simulink model "sandbox"  (R2020a)
settings: Solver=VariableStepAuto  StartTime=0.0  StopTime=2e5  RelTol=1e-3
undefined symbols (not defined in the file): agnostic_lqe_params, lqe_params, LQR_params, LQRAgnostic_params, MPC_type, MPCDiscrete_function_parameters, MPCDiscreteAgnostic_function_parameters, MPCDiscreteDiffIntegralAgnostic_function_parameters, original_lqe_params, original_LQR_params, reg
libraries: cstblocks x11
settings Model: SimulationMode=accelerator  Creator=jornbh  LastModifiedBy=jorn
settings OptimizationCC: EfficientMapNaN2IntZero=off
settings HardwareCC: TargetBitPerLong=64  TargetBitPerPointer=64  TargetBitPerSizeT=64  TargetBitPerPtrDiffT=64  TargetLongLongMode=on  TargetIntDivRoundTo=Zero  TargetEndianess=LittleEndian  TargetWordSize=64  TargetHWDeviceType=MATLAB Host  ProdEqTarget=off
settings CodeAppCC: MaxIdLength=128
settings GRTTargetCC: GRTInterface=on  UseToolchainInfoCompliant=off

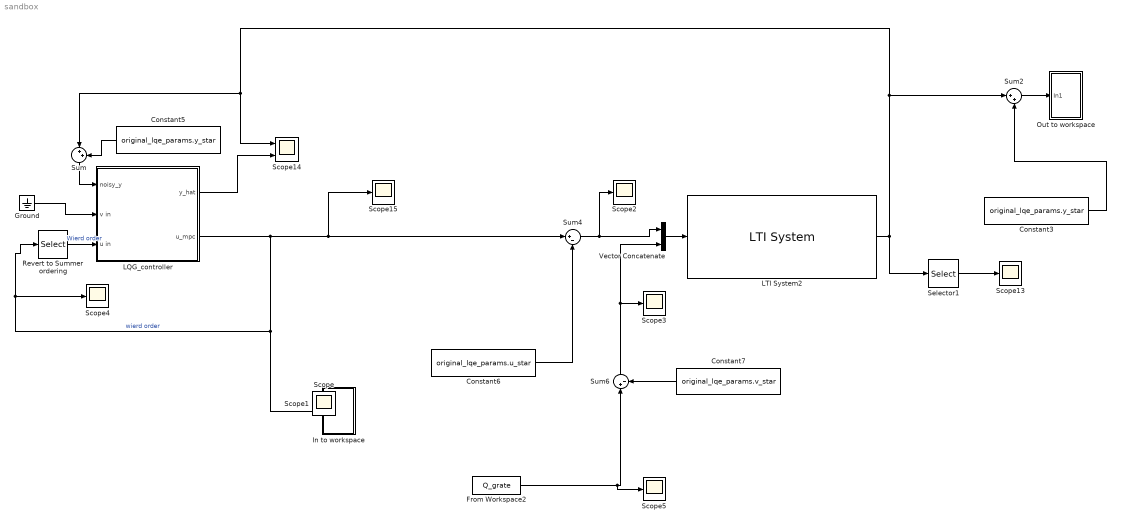
== system sandbox ==
  Constant3 : Constant  Value=original_lqe_params.y_star
  Constant5 : Constant  Value=original_lqe_params.y_star
  Constant6 : Constant  Value=original_lqe_params.u_star
  Constant7 : Constant  Value=original_lqe_params.v_star
  From Workspace2 : FromWorkspace  VariableName=Q_grate  OutputAfterFinalValue=Holding final value
  Ground : Ground
  In to workspace : Subsystem
  LQG_controller : Subsystem
  LTI System2 : cstblocks/LTI System  sys=full_estimated_plant  IC=[]
  Out to workspace : Subsystem
  Revert to Summer ordering : Selector  InputPortWidth=4  IndexOptions=Index vector (dialog)  Indices=[1 3 4 2]  OutputSizes=1
  Scope{,1..5,13,15} (8 alike) : Scope
  Scope14 : Scope  NumInputPorts=2
  Selector1 : Selector  InputPortWidth=3  IndexOptions=Index vector (dialog)  Indices=1:2  OutputSizes=1
  Sum : Sum  Inputs=|++
  Sum2 : Sum  Inputs=|++
  Sum4 : Sum  Inputs=|+-
  Sum6 : Sum  Inputs=|+-
  Vector Concatenate : Concatenate
  wires:
  LTI System2/1 -> Sum2/1, Sum/1, Scope14/1, Selector1/1
  Selector1/1 -> Scope13/1
  LQG_controller/1(y_hat) -> Scope14/2
  Ground/1 -> LQG_controller/2(v in)
  Constant3/1 -> Sum2/2
  Sum2/1 -> Out to workspace/1(In1)
  LQG_controller/2(u_mpc) -> In to workspace/1(u_mpc), Revert to Summer ordering/1, Scope4/1, Sum4/1, Scope15/1  "wierd order"
  Sum4/1 -> Scope2/1, Vector Concatenate/1
  Vector Concatenate/1 -> LTI System2/1
  Sum6/1 -> Scope3/1, Vector Concatenate/2
  Sum/1 -> LQG_controller/1(noisy_y)
  Constant5/1 -> Sum/2
  Constant6/1 -> Sum4/2
  From Workspace2/1 -> Scope5/1, Sum6/1
  Constant7/1 -> Sum6/2
  Revert to Summer ordering/1 -> LQG_controller/3(u in)  "Wierd order"

== system sandbox/In to workspace ==
  u_mpc : Inport
  Demux1 : Demux
  To Workspace4 : ToWorkspace  VariableName=simout_F_w  SaveFormat=Timeseries  SampleTime=-1
  To Workspace5 : ToWorkspace  VariableName=simout_F_aI  SaveFormat=Timeseries  SampleTime=-1
  To Workspace6 : ToWorkspace  VariableName=simout_F_aII  SaveFormat=Timeseries  SampleTime=-1
  To Workspace7 : ToWorkspace  VariableName=simout_v_grate  SaveFormat=Timeseries  SampleTime=-1
  wires:
  Demux1/3 -> To Workspace5/1
  Demux1/1 -> To Workspace6/1
  u_mpc/1 -> Demux1/1
  Demux1/2 -> To Workspace4/1
  Demux1/4 -> To Workspace7/1

== system sandbox/LQG_controller ==
  noisy_y : Inport  OutDataTypeStr=double
  v in : Inport  Port=2
  u in : Inport  Port=3
  Demux : Demux  Outputs=3
  MPC_subsystem : Subsystem
      settings: PortSchema="{\"entries\":[{\"content\":{\"sides\":[{\"content\":{\"connectorIds\":[\"In1\",\"In2\",\"In3\"]},\"type\":\"ConnectorPlacement.EquallySpacedRectSide\",\"uuid\":\"7a72dc7f-38c0-42c0-80ed-1e6801fa5538\"},{\"content\":{\"connectorIds\":[\"Out1\",\"Out2\",\"Out3\",\"Out4\",\"Out5\"],\"side\":\"RIGHT\"},\"type\":\"ConnectorPlacement.EquallySpacedRectSide\",\"uuid\":\"3b96338e-56f2-4c6d-b025-d8deebb787e0\"},{\"content\":{\"connectorIds\":[],\"side\":\"TOP\"},\"type\":\"ConnectorPlacement.EquallySpacedRectSide\",\"uuid\":\"204ca672-7e69-45d1-bd78-35e421377db1\"},{\"content\":{\"connectorIds\":[\"In4\",\"In5\"],\"side\":\"BOTTOM\"},\"type\":\"ConnectorPlacement.EquallySpacedRectSide\",\"uuid\":\"d178d855-840b-4794-a5e2-c07226929ecd\"}]},\"type\":\"ConnectorPlacement.EquallySpacedConnector\",\"uuid\":\"1be467ef-13fc-4acb-88f5-eb362f838469\"}],\"packageUris\":[\"http://schema.mathworks.com/mf0/Connector/19700101\"],\"version\":\"1.0\"}"
  Mux : Mux
  y_hat : Outport
  u_mpc : Outport  Port=2
  wires:
  u in/1 -> MPC_subsystem/4(used_inputs)
  v in/1 -> MPC_subsystem/5("\"Measured\" disturbances")
  MPC_subsystem/1(F_aII_MPC) -> Mux/1
  MPC_subsystem/2(F_aI_MPC) -> Mux/3
  MPC_subsystem/3(v_grate_MPC) -> Mux/4
  MPC_subsystem/4(F_w_MPC) -> Mux/2
  Mux/1 -> u_mpc/1
  MPC_subsystem/5(y_hat) -> y_hat/1
  Demux/2 -> MPC_subsystem/1(F_O2_in)
  Demux/1 -> MPC_subsystem/2(F_st_in)
  Demux/3 -> MPC_subsystem/3(HHV_in)
  noisy_y/1 -> Demux/1

== system sandbox/Out to workspace ==
  In1 : Inport
  Demux : Demux  Outputs=3
  To Workspace1 : ToWorkspace  VariableName=simout_HHV  SaveFormat=Timeseries  SampleTime=-1
  To Workspace2 : ToWorkspace  VariableName=simout_F_O2  SaveFormat=Timeseries  SampleTime=-1
  To Workspace3 : ToWorkspace  VariableName=simout_F_st  SaveFormat=Timeseries  SampleTime=-1
  wires:
  Demux/1 -> To Workspace3/1
  Demux/2 -> To Workspace2/1
  Demux/3 -> To Workspace1/1
  In1/1 -> Demux/1

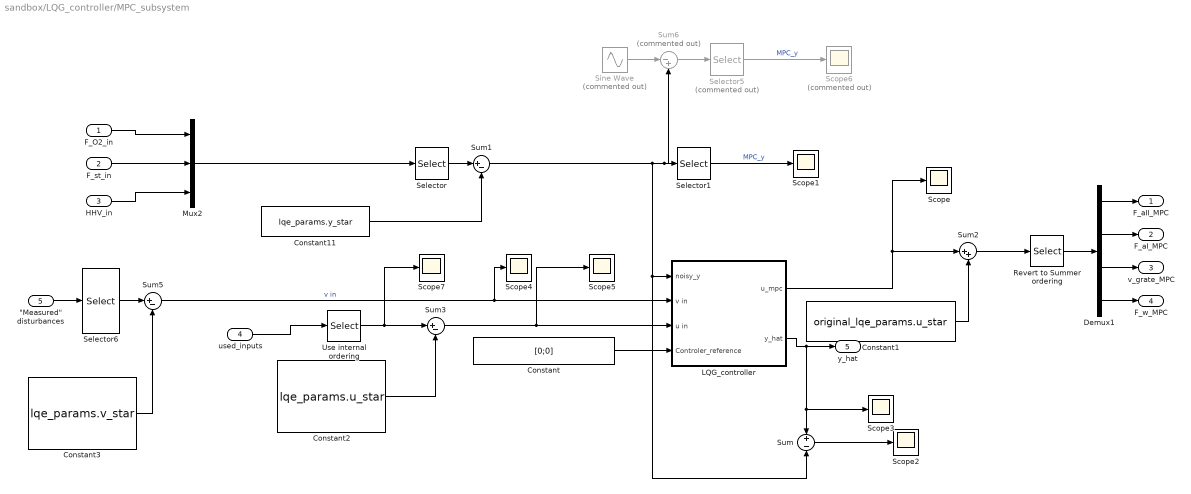
== system sandbox/LQG_controller/MPC_subsystem ==
  F_O2_in : Inport
  F_st_in : Inport  Port=2
  HHV_in : Inport  Port=3
  used_inputs : Inport  Port=4
  "\"Measured\" disturbances" : Inport  Port=5
  Constant : Constant  Value=[0;0]
  Constant1 : Constant  Value=original_lqe_params.u_star
  Constant11 : Constant  Value=lqe_params.y_star
  Constant2 : Constant  Value=lqe_params.u_star
  Constant3 : Constant  Value=lqe_params.v_star
  Demux1 : Demux
  LQG_controller : Subsystem
  Mux2 : Mux  Inputs=3
  Revert to Summer ordering : Selector  InputPortWidth=4  IndexOptions=Index vector (dialog)  Indices=[1 3 4 2]  OutputSizes=1
  Scope{,1..5,7} (7 alike) : Scope
  Scope6 : Scope  Commented=on
  Selector : Selector  InputPortWidth=3  IndexOptions=Index vector (dialog)  Indices=[2 1 3]  OutputSizes=1
  Selector1 : Selector  InputPortWidth=3  IndexOptions=Index vector (dialog)  Indices=1:2  OutputSizes=1
  Selector5 : Selector  Commented=on  InputPortWidth=3  IndexOptions=Index vector (dialog)  Indices=1:2  OutputSizes=1
  Selector6 : Selector  InputPortWidth=5  IndexOptions=Index vector (dialog)  Indices=original_lqe_params.disturbance_measurement_indecies  OutputSizes=1
  Sine Wave : Sin  Commented=on  Amplitude=reg.include_noise * 1e-3  SampleTime=0
  Sum : Sum  Inputs=+-
  Sum1 : Sum  Inputs=|+-
  Sum2 : Sum  Inputs=|++
  Sum3 : Sum  Inputs=|+-
  Sum5 : Sum  Inputs=|+-
  Sum6 : Sum  Commented=on  Inputs=|-+
  Use internal ordering : Selector  InputPortWidth=4  IndexOptions=Index vector (dialog)  Indices=[1 4 2 3]  OutputSizes=1
  F_aII_MPC : Outport
  F_aI_MPC : Outport  Port=2
  v_grate_MPC : Outport  Port=3
  F_w_MPC : Outport  Port=4
  y_hat : Outport  Port=5
  wires:
  Demux1/1 -> F_aII_MPC/1
  Demux1/3 -> v_grate_MPC/1
  Constant/1 -> LQG_controller/4(Controler_reference)
  Demux1/2 -> F_aI_MPC/1
  HHV_in/1 -> Mux2/3
  F_O2_in/1 -> Mux2/1
  F_st_in/1 -> Mux2/2
  Constant11/1 -> Sum1/2
  Demux1/4 -> F_w_MPC/1
  Sum2/1 -> Revert to Summer ordering/1
  Revert to Summer ordering/1 -> Demux1/1
  Selector/1 -> Sum1/1
  Selector1/1 -> Scope1/1  "MPC_y"
  Sum/1 -> Scope2/1
  Sum1/1 -> LQG_controller/1(noisy_y), Sum/2, Sum6/2, Selector1/1
  used_inputs/1 -> Use internal ordering/1
  Sum3/1 -> LQG_controller/3(u in), Scope5/1
  Constant2/1 -> Sum3/2
  Use internal ordering/1 -> Scope7/1, Sum3/1
  Mux2/1 -> Selector/1
  Selector5/1 -> Scope6/1  "MPC_y"
  Sine Wave/1 -> Sum6/1
  Sum6/1 -> Selector5/1
  "\"Measured\" disturbances"/1 -> Selector6/1
  Constant3/1 -> Sum5/2
  Sum5/1 -> LQG_controller/2(v in), Scope4/1  "v in"
  Selector6/1 -> Sum5/1
  Constant1/1 -> Sum2/2
  LQG_controller/2(y_hat) -> y_hat/1, Scope3/1, Sum/1
  LQG_controller/1(u_mpc) -> Scope/1, Sum2/1

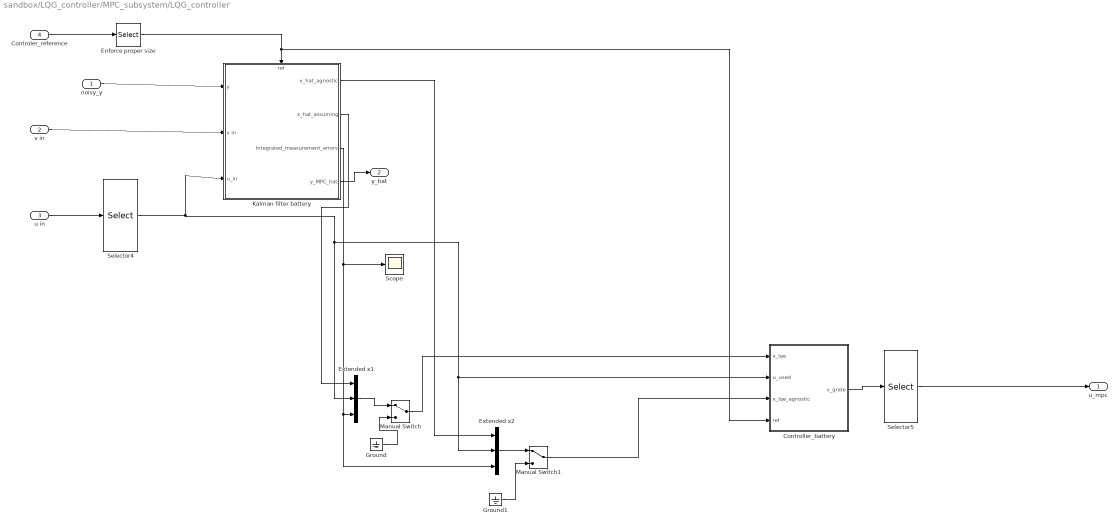
== system sandbox/LQG_controller/MPC_subsystem/LQG_controller ==
  noisy_y : Inport  OutDataTypeStr=double
  v in : Inport  Port=2
  u in : Inport  Port=3
  Controler_reference : Inport  Port=4  OutDataTypeStr=double
  Controller_battery : Subsystem
  Enforce proper size : Selector  InputPortWidth=original_LQR_params.N_refs  IndexOptions=Index vector (dialog)  Indices=1:original_LQR_params.N_refs  OutputSizes=1
  Extended x1 : Concatenate  NumInputs=3
  Extended x2 : Concatenate  NumInputs=3
  Ground : Ground
  Ground1 : Ground
  Kalman filter battery : Subsystem
      settings: PortSchema="{\"entries\":[{\"content\":{\"sides\":[{\"content\":{\"connectorIds\":[\"In1\",\"In2\",\"In3\"]},\"type\":\"ConnectorPlacement.EquallySpacedRectSide\",\"uuid\":\"1c993a74-2ebc-4ff1-8a36-810b6615b91b\"},{\"content\":{\"connectorIds\":[\"Out1\",\"Out2\",\"Out3\",\"Out4\"],\"side\":\"RIGHT\"},\"type\":\"ConnectorPlacement.EquallySpacedRectSide\",\"uuid\":\"f47ce850-e8b0-4437-a8da-01c6ea316d70\"},{\"content\":{\"connectorIds\":[],\"side\":\"TOP\"},\"type\":\"ConnectorPlacement.EquallySpacedRectSide\",\"uuid\":\"49075f58-3726-424f-842a-93e04b24d953\"},{\"content\":{\"connectorIds\":[\"In4\"],\"side\":\"BOTTOM\"},\"type\":\"ConnectorPlacement.EquallySpacedRectSide\",\"uuid\":\"0a8cab2c-6cc5-4573-a1bf-983f74a1ee29\"}]},\"type\":\"ConnectorPlacement.EquallySpacedConnector\",\"uuid\":\"113553bc-ba05-4a25-98d3-042b5b48218e\"}],\"packageUris\":[\"http://schema.mathworks.com/mf0/Connector/19700101\"],\"version\":\"1.0\"}"
  Manual Switch : ManualSwitch
  Manual Switch1 : ManualSwitch
  Scope : Scope
  Selector4 : Selector  InputPortWidth=4  IndexOptions=Index vector (dialog)  Indices=1:4  OutputSizes=1
  Selector5 : Selector  InputPortWidth=4  IndexOptions=Index vector (dialog)  Indices=1:4  OutputSizes=1
  u_mpc : Outport
  y_hat : Outport  Port=2
  wires:
  Controler_reference/1 -> Enforce proper size/1
  u in/1 -> Selector4/1
  Enforce proper size/1 -> Controller_battery/4(ref), Kalman filter battery/4(ref)
  Kalman filter battery/2(Integrated_measurement_errors) -> Extended x2/3, Extended x1/3, Scope/1
  noisy_y/1 -> Kalman filter battery/3(y)
  Kalman filter battery/1(y_MPC_hat) -> y_hat/1
  Selector5/1 -> u_mpc/1
  Selector4/1 -> Extended x1/2, Extended x2/2, Controller_battery/2(u_used), Kalman filter battery/1(u_in)
  Controller_battery/1(v_grate) -> Selector5/1
  v in/1 -> Kalman filter battery/2(v in)
  Kalman filter battery/4(x_hat_agnostic) -> Extended x2/1
  Manual Switch/1 -> Controller_battery/1(x_lqe)
  Manual Switch1/1 -> Controller_battery/3(x_lqe_agnostic)
  Kalman filter battery/3(x_hat_assuming) -> Extended x1/1
  Extended x1/1 -> Manual Switch/1
  Extended x2/1 -> Manual Switch1/1
  Ground/1 -> Manual Switch/2
  Ground1/1 -> Manual Switch1/2

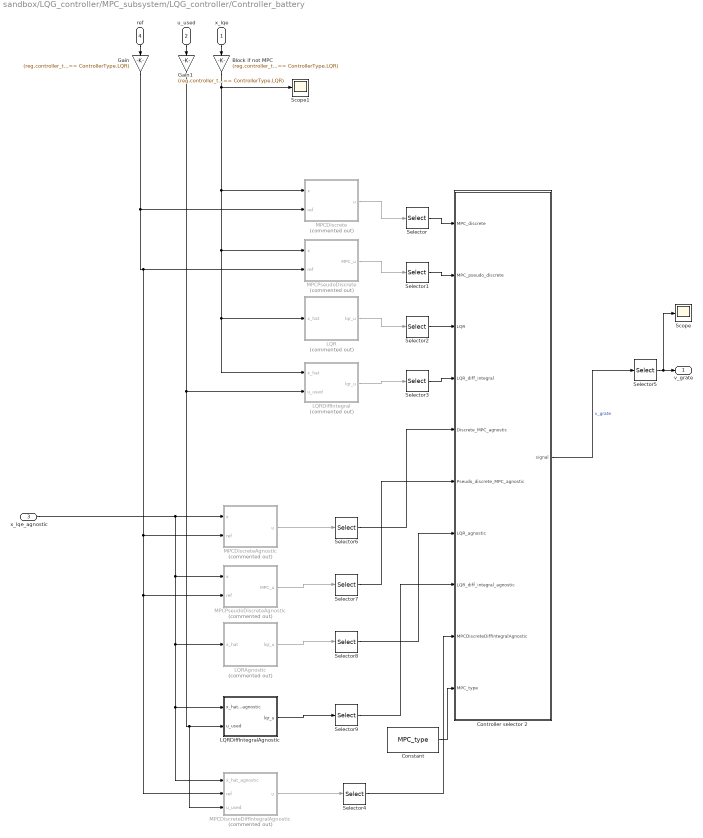
== system sandbox/LQG_controller/MPC_subsystem/LQG_controller/Controller_battery ==
  x_lqe : Inport
  u_used : Inport  Port=2
  x_lqe_agnostic : Inport  Port=3
  ref : Inport  Port=4
  Block if not MPC : Gain  Gain=(reg.controller_type == ControllerType.MPC)|| (reg.controller_type == ControllerType.LQR)
  Constant : Constant  Value=MPC_type
  Controller selector 2 : MATLAB Function  TreatAsAtomicUnit=on
  Gain : Gain  Gain=(reg.controller_type == ControllerType.MPC)|| (reg.controller_type == ControllerType.LQR)
  Gain1 : Gain  Gain=(reg.controller_type == ControllerType.MPC)|| (reg.controller_type == ControllerType.LQR)
  LQR : Subsystem  Commented=on
  LQRAgnostic : Subsystem  Commented=on
  LQRDiffIntegral : Subsystem  Commented=on
  LQRDiffIntegralAgnostic : Subsystem
  MPCDiscrete : Subsystem  Commented=on
  MPCDiscreteAgnostic : Subsystem  Commented=on
  MPCDiscreteDiffIntegralAgnostic : Subsystem  Commented=on
  MPCPseudoDiscrete : Subsystem  Commented=on
  MPCPseudoDiscreteAgnostic : Subsystem  Commented=on
  Scope : Scope
  Scope1 : Scope
  Selector{,1..9} (10 alike) : Selector  InputPortWidth=4  IndexOptions=Index vector (dialog)  Indices=1:4  OutputSizes=1
  v_grate : Outport
  wires:
  MPCPseudoDiscrete/1(MPC_u) -> Selector1/1
  LQR/1(lqr_u) -> Selector2/1
  MPCDiscrete/1(u) -> Selector/1
  LQRDiffIntegral/1(lqr_u) -> Selector3/1
  Controller selector 2/1(signal) -> Selector5/1  "v_grate"
  u_used/1 -> Gain1/1
  ref/1 -> Gain/1
  x_lqe/1 -> Block if not MPC/1
  Selector/1 -> Controller selector 2/1(MPC_discrete)
  Selector1/1 -> Controller selector 2/2(MPC_pseudo_discrete)
  Selector2/1 -> Controller selector 2/3(LQR)
  Selector3/1 -> Controller selector 2/4(LQR_diff_integral)
  Constant/1 -> Controller selector 2/10(MPC_type)
  Selector5/1 -> Scope/1, v_grate/1
  MPCDiscreteAgnostic/1(u) -> Selector6/1
  LQRDiffIntegralAgnostic/1(lqr_u) -> Selector9/1
  LQRAgnostic/1(lqr_u) -> Selector8/1
  MPCPseudoDiscreteAgnostic/1(MPC_u) -> Selector7/1
  Selector6/1 -> Controller selector 2/5(Discrete_MPC_agnostic)
  Selector9/1 -> Controller selector 2/8(LQR_diff_integral_agnostic)
  Selector7/1 -> Controller selector 2/6(Pseudo_discrete_MPC_agnostic)
  Selector8/1 -> Controller selector 2/7(LQR_agnostic)
  Gain/1 -> MPCDiscreteDiffIntegralAgnostic/2(ref), MPCPseudoDiscreteAgnostic/2(ref), MPCDiscreteAgnostic/2(ref), MPCPseudoDiscrete/2(ref), MPCDiscrete/2(ref)
  Block if not MPC/1 -> Scope1/1, LQRDiffIntegral/1(x_hat), LQR/1(x_hat), MPCPseudoDiscrete/1(x), MPCDiscrete/1(x)
  x_lqe_agnostic/1 -> MPCPseudoDiscreteAgnostic/1(x), LQRAgnostic/1(x_hat), MPCDiscreteDiffIntegralAgnostic/1(x_hat_agnostic), LQRDiffIntegralAgnostic/1(x_hat_agnostic), MPCDiscreteAgnostic/1(x)
  MPCDiscreteDiffIntegralAgnostic/1(u) -> Selector4/1
  Selector4/1 -> Controller selector 2/9(MPCDiscreteDiffIntegralAgnostic)
  Gain1/1 -> MPCDiscreteDiffIntegralAgnostic/3(u_used), LQRDiffIntegralAgnostic/2(u_used), LQRDiffIntegral/2(u_used)

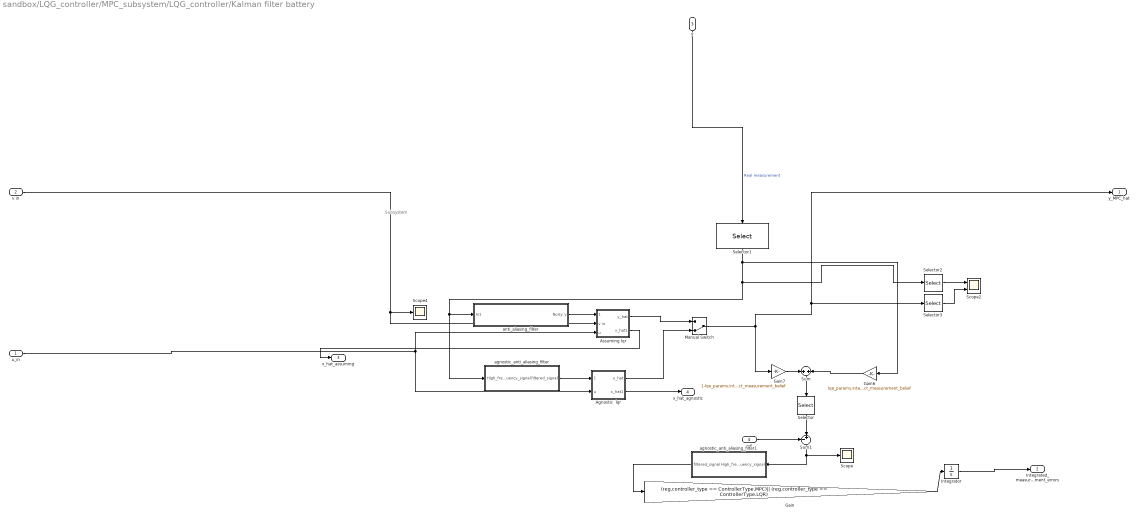
== system sandbox/LQG_controller/MPC_subsystem/LQG_controller/Kalman filter battery ==
  note: Subsystem
  u_in : Inport
  v in : Inport  Port=2
  y : Inport  Port=3
  ref : Inport  Port=4
  Agnostic  lqr : Subsystem
  Assuming lqr : Subsystem
  Gain : Gain  Gain=(reg.controller_type == ControllerType.MPC)|| (reg.controller_type == ControllerType.LQR)
  Gain6 : Gain  Gain=lqe_params.integrator_direct_measurement_belief
  Gain7 : Gain  Gain=1-lqe_params.integrator_direct_measurement_belief
  Integrator : Integrator
  Manual Switch : ManualSwitch  CurrentSetting=0
  Scope : Scope
  Scope2 : Scope  NumInputPorts=2
  Scope4 : Scope
  Selector : Selector  InputPortWidth=3  IndexOptions=Index vector (dialog)  Indices=1:2  OutputSizes=1
  Selector1 : Selector  InputPortWidth=3  IndexOptions=Index vector (dialog)  Indices=1:3  OutputSizes=1
  Selector2 : Selector  InputPortWidth=3  IndexOptions=Index vector (dialog)  Indices=1:2  OutputSizes=1
  Selector3 : Selector  InputPortWidth=3  IndexOptions=Index vector (dialog)  Indices=1:2  OutputSizes=1
  Sum : Sum
  Sum1 : Sum  Inputs=-+|
  agnostic_anti_aliasing_filter : Subsystem
  agnostic_anti_aliasing_filter1 : Subsystem
  anti_aliasing_filter : Subsystem
  y_MPC_hat : Outport
  Integrated_measurement_errors : Outport  Port=2
  x_hat_assuming : Outport  Port=3
  x_hat_agnostic : Outport  Port=4
  wires:
  y/1 -> Selector1/1  "Real measurement"
  Manual Switch/1 -> y_MPC_hat/1, Selector3/1, Gain7/1
  Integrator/1 -> Integrated_measurement_errors/1
  Assuming lqr/2(x_hat1) -> x_hat_assuming/1
  Agnostic  lqr/2(x_hat1) -> x_hat_agnostic/1
  Selector/1 -> Sum1/2
  Gain/1 -> Integrator/1
  Assuming lqr/1(y_hat) -> Manual Switch/1
  u_in/1 -> Agnostic  lqr/2(u), Assuming lqr/3(u)
  Gain7/1 -> Sum/1
  ref/1 -> Sum1/1
  Selector1/1 -> anti_aliasing_filter/1(In1), agnostic_anti_aliasing_filter/1(High_frequency_signal), Selector2/1, Gain6/1
  Sum1/1 -> Scope/1, agnostic_anti_aliasing_filter1/1(High_frequency_signal)
  Selector2/1 -> Scope2/1
  v in/1 -> Assuming lqr/2(v in), Scope4/1
  Agnostic  lqr/1(y_hat) -> Manual Switch/2
  Sum/1 -> Selector/1
  Selector3/1 -> Scope2/2
  anti_aliasing_filter/1(Noisy y) -> Assuming lqr/1(Noisy y)
  Gain6/1 -> Sum/2
  agnostic_anti_aliasing_filter/1(filtered_signal) -> Agnostic  lqr/1(Noisy y)
  agnostic_anti_aliasing_filter1/1(filtered_signal) -> Gain/1

== system sandbox/LQG_controller/MPC_subsystem/LQG_controller/Controller_battery/LQR ==
  x_hat : Inport
  LQR : Gain  Gain=-LQR_params.K_lqr  Multiplication=Matrix(K*u)
  LTI System1 : cstblocks/LTI System  sys=original_LQR_params.input_filter  IC=[]
  Scope1 : Scope
  Scope2 : Scope
  lqr_u : Outport
  wires:
  LQR/1 -> LTI System1/1  "lqr_u"
  x_hat/1 -> Scope1/1, LQR/1
  LTI System1/1 -> Scope2/1, lqr_u/1

== system sandbox/LQG_controller/MPC_subsystem/LQG_controller/Controller_battery/LQRAgnostic ==
  x_hat : Inport
  LQR : Gain  Gain=-LQRAgnostic_params.K_lqr  Multiplication=Matrix(K*u)
  LTI System1 : cstblocks/LTI System  sys=original_LQRAgnostic_params.input_filter  IC=[]
  Scope1 : Scope
  Scope2 : Scope
  lqr_u : Outport
  wires:
  LTI System1/1 -> Scope2/1, lqr_u/1
  x_hat/1 -> LQR/1, Scope1/1
  LQR/1 -> LTI System1/1  "lqr_u"

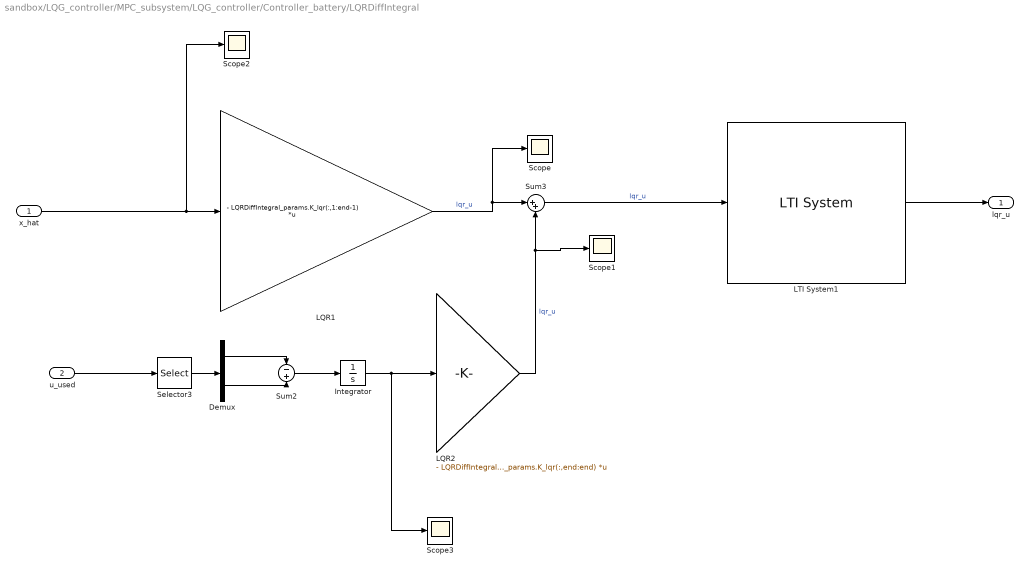
== system sandbox/LQG_controller/MPC_subsystem/LQG_controller/Controller_battery/LQRDiffIntegral ==
  x_hat : Inport
  u_used : Inport  Port=2
  Demux : Demux  Outputs=2
  Integrator : Integrator
  LQR1 : Gain  Gain=- LQRDiffIntegral_params.K_lqr(:,1:end-1)  Multiplication=Matrix(K*u)
  LQR2 : Gain  Gain=- LQRDiffIntegral_params.K_lqr(:,end:end)  Multiplication=Matrix(K*u)
  LTI System1 : cstblocks/LTI System  sys=original_LQRDiffIntegral_params.input_filter  IC=[]
  Scope{,1..3} (4 alike) : Scope
  Selector3 : Selector  InputPortWidth=4  IndexOptions=Index vector (dialog)  Indices=[1 3]  OutputSizes=1
  Sum2 : Sum  Inputs=-+
  Sum3 : Sum  Inputs=|++
  lqr_u : Outport
  wires:
  LQR1/1 -> Scope/1, Sum3/1  "lqr_u"
  u_used/1 -> Selector3/1
  Sum3/1 -> LTI System1/1  "lqr_u"
  Sum2/1 -> Integrator/1
  Demux/2 -> Sum2/2
  Integrator/1 -> Scope3/1, LQR2/1
  Selector3/1 -> Demux/1
  Demux/1 -> Sum2/1
  x_hat/1 -> Scope2/1, LQR1/1
  LQR2/1 -> Scope1/1, Sum3/2  "lqr_u"
  LTI System1/1 -> lqr_u/1

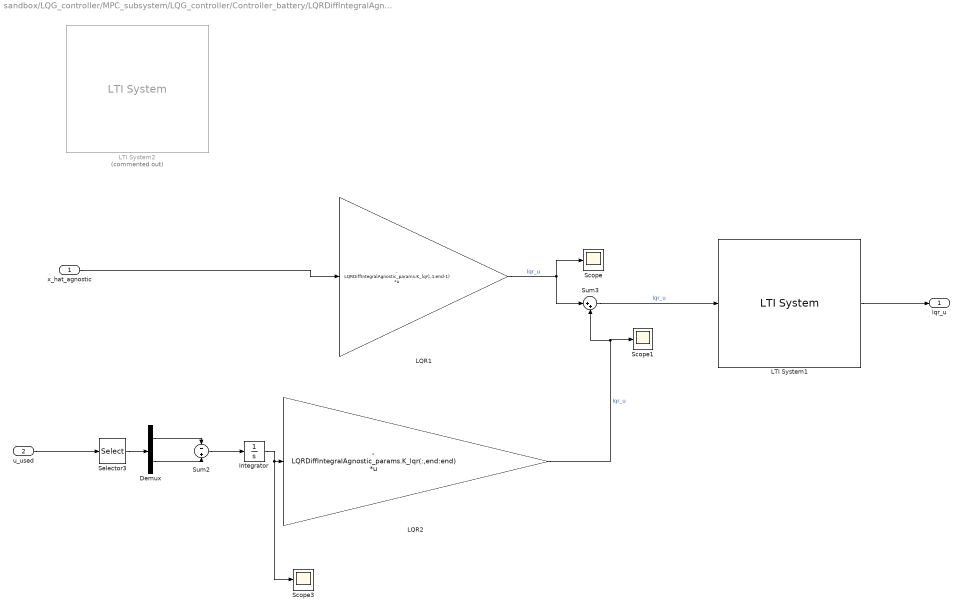
== system sandbox/LQG_controller/MPC_subsystem/LQG_controller/Controller_battery/LQRDiffIntegralAgnostic ==
  x_hat_agnostic : Inport
  u_used : Inport  Port=2
  Demux : Demux  Outputs=2
  Integrator : Integrator
  LQR1 : Gain  Gain=- LQRDiffIntegralAgnostic_params.K_lqr(:,1:end-1)  Multiplication=Matrix(K*u)
  LQR2 : Gain  Gain=- LQRDiffIntegralAgnostic_params.K_lqr(:,end:end)  Multiplication=Matrix(K*u)
  LTI System1 : cstblocks/LTI System  sys=original_LQRDiffIntegralAgnostic_params.input_filter  IC=[]
  LTI System2 : cstblocks/LTI System  Commented=on  sys=original_diff_agnostic_mpc_params.input_filter  IC=[]
  Scope : Scope
  Scope1 : Scope
  Scope3 : Scope
  Selector3 : Selector  InputPortWidth=4  IndexOptions=Index vector (dialog)  Indices=[1 3]  OutputSizes=1
  Sum2 : Sum  Inputs=-+
  Sum3 : Sum  Inputs=|++
  lqr_u : Outport
  wires:
  LQR2/1 -> Sum3/2, Scope1/1  "lqr_u"
  Demux/1 -> Sum2/1
  Selector3/1 -> Demux/1
  Integrator/1 -> Scope3/1, LQR2/1
  Demux/2 -> Sum2/2
  Sum2/1 -> Integrator/1
  Sum3/1 -> LTI System1/1  "lqr_u"
  LQR1/1 -> Sum3/1, Scope/1  "lqr_u"
  LTI System1/1 -> lqr_u/1
  x_hat_agnostic/1 -> LQR1/1
  u_used/1 -> Selector3/1

== system sandbox/LQG_controller/MPC_subsystem/LQG_controller/Controller_battery/MPCDiscrete ==
  x : Inport
  ref : Inport  Port=2
  LTI System1 : cstblocks/LTI System  sys=original_MPCDiscrete_params .input_filter  IC=[]
  MATLAB Function : MATLAB Function  TreatAsAtomicUnit=on
  Memory1 : Memory  InitialCondition=MPCDiscrete_function_parameters.iA  InheritSampleTime=on  LinearizeMemory=on  LinearizeAsDelay=on
  Memory4 : Memory  InheritSampleTime=on  LinearizeMemory=on  LinearizeAsDelay=on
  u : Outport
  wires:
  Memory4/1 -> MATLAB Function/3(u_prev)
  MATLAB Function/2(new_iA) -> Memory1/1
  MATLAB Function/1(u) -> LTI System1/1, Memory4/1
  Memory1/1 -> MATLAB Function/4(iA)
  ref/1 -> MATLAB Function/2(ref)
  x/1 -> MATLAB Function/1(x)
  LTI System1/1 -> u/1

== system sandbox/LQG_controller/MPC_subsystem/LQG_controller/Controller_battery/MPCDiscreteAgnostic ==
  x : Inport
  ref : Inport  Port=2
  LTI System1 : cstblocks/LTI System  sys=original_MPCDiscreteAgnostic_params.input_filter  IC=[]
  MATLAB Function : MATLAB Function  TreatAsAtomicUnit=on
  Memory1 : Memory  InitialCondition=MPCDiscreteAgnostic_function_parameters.iA  InheritSampleTime=on  LinearizeMemory=on  LinearizeAsDelay=on
  Memory4 : Memory  InheritSampleTime=on  LinearizeMemory=on  LinearizeAsDelay=on
  u : Outport
  wires:
  LTI System1/1 -> u/1
  x/1 -> MATLAB Function/1(x)
  ref/1 -> MATLAB Function/2(ref)
  Memory1/1 -> MATLAB Function/4(iA)
  MATLAB Function/1(u) -> Memory4/1, LTI System1/1
  MATLAB Function/2(new_iA) -> Memory1/1
  Memory4/1 -> MATLAB Function/3(u_prev)

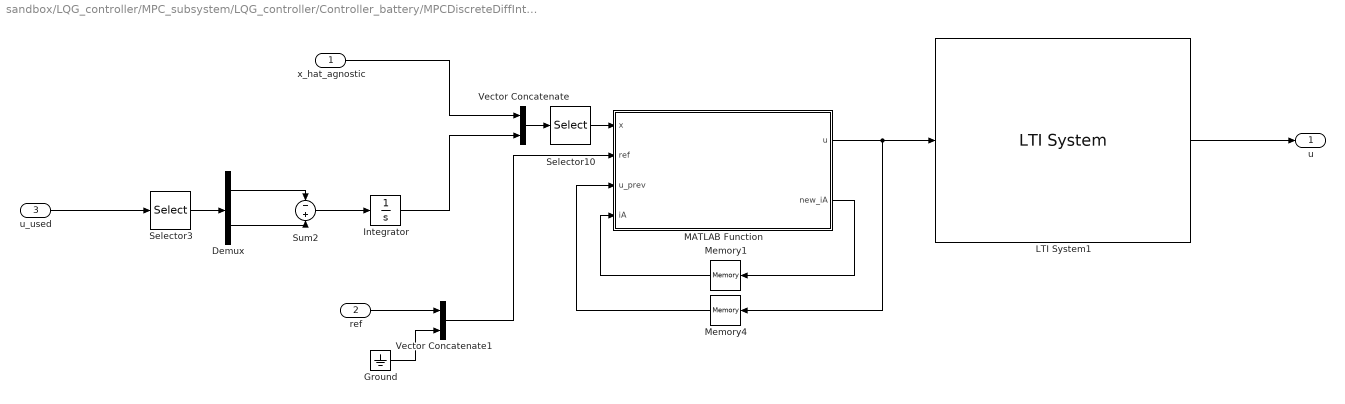
== system sandbox/LQG_controller/MPC_subsystem/LQG_controller/Controller_battery/MPCDiscreteDiffIntegralAgnostic ==
  x_hat_agnostic : Inport
  ref : Inport  Port=2
  u_used : Inport  Port=3
  Demux : Demux  Outputs=2
  Ground : Ground
  Integrator : Integrator
  LTI System1 : cstblocks/LTI System  sys=original_MPCDiscreteAgnostic_params.input_filter  IC=[]
  MATLAB Function : MATLAB Function  TreatAsAtomicUnit=on
  Memory1 : Memory  InitialCondition=MPCDiscreteDiffIntegralAgnostic_function_parameters.iA  InheritSampleTime=on  LinearizeMemory=on  LinearizeAsDelay=on
  Memory4 : Memory  InheritSampleTime=on  LinearizeMemory=on  LinearizeAsDelay=on
  Selector10 : Selector  InputPortWidth=19  IndexOptions=Index vector (dialog)  Indices=1:19  OutputSizes=1
  Selector3 : Selector  InputPortWidth=4  IndexOptions=Index vector (dialog)  Indices=[1 3]  OutputSizes=1
  Sum2 : Sum  Inputs=-+
  Vector Concatenate : Concatenate
  Vector Concatenate1 : Concatenate
  u : Outport
  wires:
  LTI System1/1 -> u/1
  x_hat_agnostic/1 -> Vector Concatenate/1
  Vector Concatenate1/1 -> MATLAB Function/2(ref)
  Memory1/1 -> MATLAB Function/4(iA)
  MATLAB Function/1(u) -> Memory4/1, LTI System1/1
  MATLAB Function/2(new_iA) -> Memory1/1
  Memory4/1 -> MATLAB Function/3(u_prev)
  Selector3/1 -> Demux/1
  Demux/1 -> Sum2/1
  u_used/1 -> Selector3/1
  Demux/2 -> Sum2/2
  Sum2/1 -> Integrator/1
  Integrator/1 -> Vector Concatenate/2
  Vector Concatenate/1 -> Selector10/1
  Selector10/1 -> MATLAB Function/1(x)
  ref/1 -> Vector Concatenate1/1
  Ground/1 -> Vector Concatenate1/2

== system sandbox/LQG_controller/MPC_subsystem/LQG_controller/Controller_battery/MPCPseudoDiscrete ==
  x : Inport
  ref : Inport  Port=2
  Cont mpc : MATLAB Function
  LTI System1 : cstblocks/LTI System  sys=original_MPCPseudoDiscrete_params.input_filter  IC=[]
  MPC_u : Outport
  wires:
  Cont mpc/1(u) -> LTI System1/1  "MPC_u"
  x/1 -> Cont mpc/1(x)
  ref/1 -> Cont mpc/2(ref)
  LTI System1/1 -> MPC_u/1

== system sandbox/LQG_controller/MPC_subsystem/LQG_controller/Controller_battery/MPCPseudoDiscreteAgnostic ==
  x : Inport
  ref : Inport  Port=2
  Cont mpc : MATLAB Function
  LTI System1 : cstblocks/LTI System  sys=original_MPCPseudoDiscreteAgnostic_params.input_filter  IC=[]
  MPC_u : Outport
  wires:
  LTI System1/1 -> MPC_u/1
  ref/1 -> Cont mpc/2(ref)
  x/1 -> Cont mpc/1(x)
  Cont mpc/1(u) -> LTI System1/1  "MPC_u"

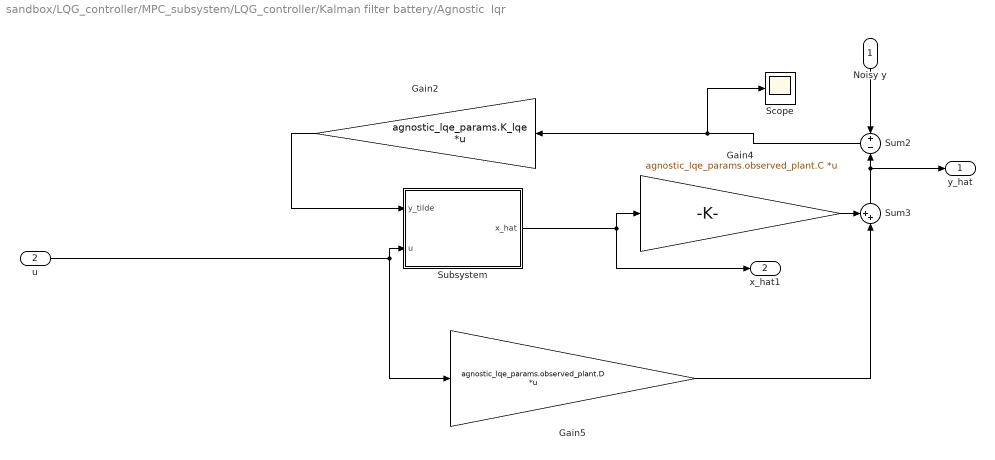
== system sandbox/LQG_controller/MPC_subsystem/LQG_controller/Kalman filter battery/Agnostic  lqr ==
  Noisy y : Inport
  u : Inport  Port=2
  Gain2 : Gain  Gain=agnostic_lqe_params.K_lqe  Multiplication=Matrix(K*u)
  Gain4 : Gain  Gain=agnostic_lqe_params.observed_plant.C  Multiplication=Matrix(K*u)
  Gain5 : Gain  Gain=agnostic_lqe_params.observed_plant.D  Multiplication=Matrix(K*u)
  Scope : Scope
  Subsystem : Subsystem
  Sum2 : Sum  Inputs=+-
  Sum3 : Sum  Inputs=++|
  y_hat : Outport
  x_hat1 : Outport  Port=2
  wires:
  Noisy y/1 -> Sum2/1
  Gain5/1 -> Sum3/2
  Gain4/1 -> Sum3/1
  Sum2/1 -> Gain2/1, Scope/1
  u/1 -> Gain5/1, Subsystem/2(u)
  Sum3/1 -> y_hat/1, Sum2/2
  Subsystem/1(x_hat) -> Gain4/1, x_hat1/1
  Gain2/1 -> Subsystem/1(y_tilde)

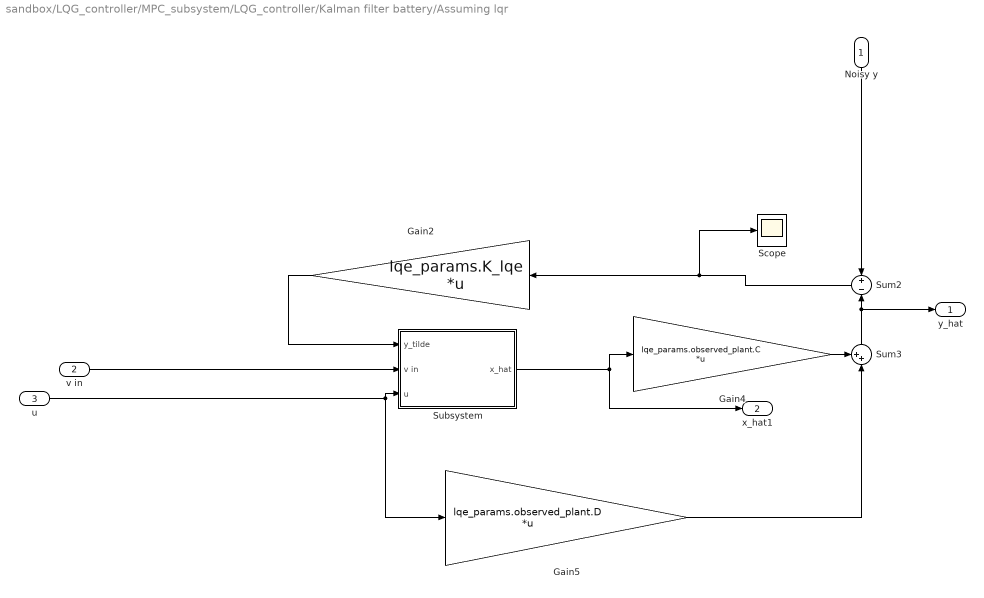
== system sandbox/LQG_controller/MPC_subsystem/LQG_controller/Kalman filter battery/Assuming lqr ==
  Noisy y : Inport
  v in : Inport  Port=2
  u : Inport  Port=3
  Gain2 : Gain  Gain=lqe_params.K_lqe  Multiplication=Matrix(K*u)
  Gain4 : Gain  Gain=lqe_params.observed_plant.C  Multiplication=Matrix(K*u)
  Gain5 : Gain  Gain=lqe_params.observed_plant.D  Multiplication=Matrix(K*u)
  Scope : Scope
  Subsystem : Subsystem
  Sum2 : Sum  Inputs=+-
  Sum3 : Sum  Inputs=++|
  y_hat : Outport
  x_hat1 : Outport  Port=2
  wires:
  Gain2/1 -> Subsystem/1(y_tilde)
  Subsystem/1(x_hat) -> x_hat1/1, Gain4/1
  Sum3/1 -> Sum2/2, y_hat/1
  u/1 -> Subsystem/3(u), Gain5/1
  Sum2/1 -> Scope/1, Gain2/1
  Gain4/1 -> Sum3/1
  Gain5/1 -> Sum3/2
  Noisy y/1 -> Sum2/1
  v in/1 -> Subsystem/2(v in)

== system sandbox/LQG_controller/MPC_subsystem/LQG_controller/Kalman filter battery/agnostic_anti_aliasing_filter ==
  High_frequency_signal : Inport
  Gain1 : Gain  Gain=agnostic_lqe_params.anti_aliasing_filter.B  Multiplication=Matrix(K*u)
  Gain2 : Gain  Gain=agnostic_lqe_params.anti_aliasing_filter.A  Multiplication=Matrix(K*u)
  Gain3 : Gain  Gain=agnostic_lqe_params.anti_aliasing_filter.C  Multiplication=Matrix(K*u)
  Integrator1 : Integrator
  Sum2 : Sum  Inputs=|++
  filtered_signal : Outport
  wires:
  Integrator1/1 -> Gain2/1, Gain3/1
  Sum2/1 -> Integrator1/1
  High_frequency_signal/1 -> Gain1/1
  Gain3/1 -> filtered_signal/1
  Gain1/1 -> Sum2/1
  Gain2/1 -> Sum2/2

== system sandbox/LQG_controller/MPC_subsystem/LQG_controller/Kalman filter battery/agnostic_anti_aliasing_filter1 ==
  High_frequency_signal : Inport
  Gain1 : Gain  Gain=agnostic_lqe_params.anti_aliasing_filter.B*eye(3,2)  Multiplication=Matrix(K*u)
  Gain2 : Gain  Gain=agnostic_lqe_params.anti_aliasing_filter.A  Multiplication=Matrix(K*u)
  Gain3 : Gain  Gain=eye(2,3)*agnostic_lqe_params.anti_aliasing_filter.C  Multiplication=Matrix(K*u)
  Integrator1 : Integrator
  Sum2 : Sum  Inputs=|++
  filtered_signal : Outport
  wires:
  Gain2/1 -> Sum2/2
  Gain1/1 -> Sum2/1
  Gain3/1 -> filtered_signal/1
  High_frequency_signal/1 -> Gain1/1
  Sum2/1 -> Integrator1/1
  Integrator1/1 -> Gain3/1, Gain2/1

== system sandbox/LQG_controller/MPC_subsystem/LQG_controller/Kalman filter battery/anti_aliasing_filter ==
  In1 : Inport
  Gain1 : Gain  Gain=lqe_params.anti_aliasing_filter.B  Multiplication=Matrix(K*u)
  Gain2 : Gain  Gain=lqe_params.anti_aliasing_filter.A  Multiplication=Matrix(K*u)
  Gain3 : Gain  Gain=lqe_params.anti_aliasing_filter.B  Multiplication=Matrix(K*u)
  Integrator1 : Integrator
  Sum2 : Sum  Inputs=|++
  Noisy y : Outport
  wires:
  Gain1/1 -> Sum2/1
  Gain2/1 -> Sum2/2
  Sum2/1 -> Integrator1/1
  Integrator1/1 -> Gain2/1, Gain3/1
  In1/1 -> Gain1/1
  Gain3/1 -> Noisy y/1

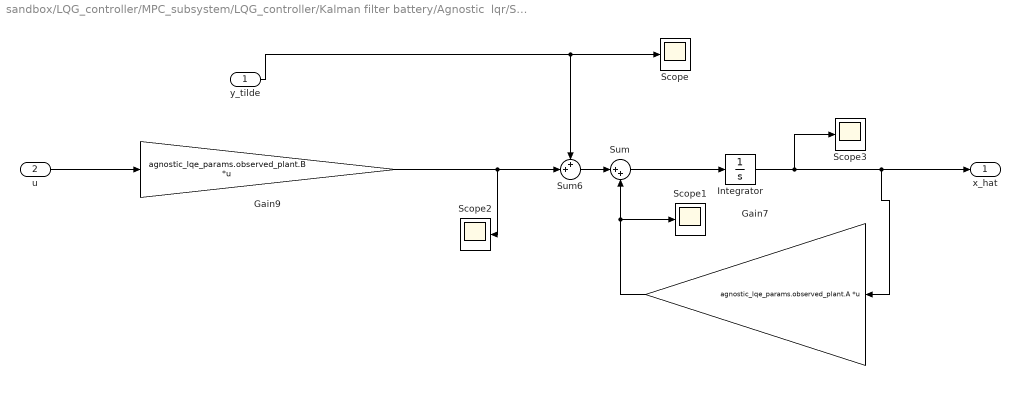
== system sandbox/LQG_controller/MPC_subsystem/LQG_controller/Kalman filter battery/Agnostic  lqr/Subsystem ==
  y_tilde : Inport
  u : Inport  Port=2
  Gain7 : Gain  Gain=agnostic_lqe_params.observed_plant.A  Multiplication=Matrix(K*u)
  Gain9 : Gain  Gain=agnostic_lqe_params.observed_plant.B  Multiplication=Matrix(K*u)
  Integrator : Integrator
  Scope{,1..3} (4 alike) : Scope
  Sum : Sum  Inputs=|++
  Sum6 : Sum  Inputs=++|
  x_hat : Outport
  wires:
  u/1 -> Gain9/1
  y_tilde/1 -> Sum6/1, Scope/1
  Integrator/1 -> Scope3/1, Gain7/1, x_hat/1
  Sum6/1 -> Sum/1
  Sum/1 -> Integrator/1
  Gain7/1 -> Sum/2, Scope1/1
  Gain9/1 -> Scope2/1, Sum6/2

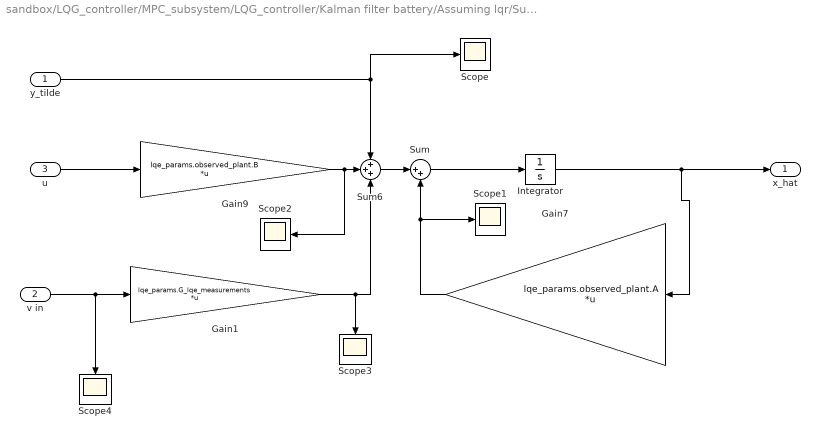
== system sandbox/LQG_controller/MPC_subsystem/LQG_controller/Kalman filter battery/Assuming lqr/Subsystem ==
  y_tilde : Inport
  v in : Inport  Port=2
  u : Inport  Port=3
  Gain1 : Gain  Gain=lqe_params.G_lqe_measurements  Multiplication=Matrix(K*u)
  Gain7 : Gain  Gain=lqe_params.observed_plant.A  Multiplication=Matrix(K*u)
  Gain9 : Gain  Gain=lqe_params.observed_plant.B  Multiplication=Matrix(K*u)
  Integrator : Integrator
  Scope{,1..4} (5 alike) : Scope
  Sum : Sum  Inputs=|++
  Sum6 : Sum  Inputs=+++
  x_hat : Outport
  wires:
  Gain7/1 -> Scope1/1, Sum/2
  Sum/1 -> Integrator/1
  Gain9/1 -> Scope2/1, Sum6/2
  Sum6/1 -> Sum/1
  Integrator/1 -> x_hat/1, Gain7/1
  y_tilde/1 -> Sum6/1, Scope/1
  u/1 -> Gain9/1
  v in/1 -> Scope4/1, Gain1/1
  Gain1/1 -> Scope3/1, Sum6/3

== matlab function sandbox/LQG_controller/MPC_subsystem/LQG_controller/Controller_battery/Controller selector 2 ==
  data: MPC_discrete input; MPC_pseudo_discrete input; signal output; LQR input; LQR_diff_integral input; Discrete_MPC_agnostic input; Pseudo_discrete_MPC_agnostic input; LQR_agnostic input; LQR_diff_integral_agnostic input; MPCDiscreteDiffIntegralAgnostic input; MPC_type input
function signal = ChooseMPCType(MPC_discrete,MPC_pseudo_discrete, LQR, LQR_diff_integral,Discrete_MPC_agnostic, Pseudo_discrete_MPC_agnostic, LQR_agnostic, LQR_diff_integral_agnostic, MPCDiscreteDiffIntegralAgnostic, MPC_type)
   
switch(MPC_type)
        % Assuming inputs
        case MPCType.MPCDiscrete
            signal = MPC_discrete;
        case MPCType.MPCPseudoDiscrete
            signal = MPC_pseudo_discrete;
        case MPCType.LQR
            signal = LQR;
        case MPCType.LQRDiffIntegral
            signal = LQR_diff_integral; 
            
        % Agnostic inputs
        case MPCType.MPCDiscreteAgnostic
            signal = Discrete_MPC_agnostic;
        case MPCType.MPCPseudoDiscreteAgnostic
            signal =Pseudo_discrete_MPC_agnostic;
        case MPCType.LQRAgnostic
            signal = LQR_agnostic;
        case MPCType.LQRDiffIntegralAgnostic
            signal = LQR_diff_integral_agnostic; 
    otherwise
        signal = MPCDiscreteDiffIntegralAgnostic; 
    end
end

== matlab function sandbox/LQG_controller/MPC_subsystem/LQG_controller/Controller_battery/MPCDiscrete/MATLAB Function ==
  settings: updateMethod=DISCRETE  sampleTime=MPCDiscrete_params.MPC_plant.Ts
  data: x input; ref input; u_prev input; iA input; u output size=4; MPCDiscrete_function_parameters parameter; new_iA output
function [u, new_iA] = fcn(x, ref, u_prev, iA,...
    MPCDiscrete_function_parameters)


% Discrete_MPC_function_parameter
   % Might just set these manually... 
    MPC_opt = mpcActiveSetOptions;
    MPC_opt.IntegrityChecks = false;
    MPC_opt.UseHessianAsInput = false; 

%% Uncertain part
    new_b0 = MPCDiscrete_function_parameters.b0;
    
    F = (                                           ...
                (MPCDiscrete_function_parameters.F_y_ref* ref)           ...
            +    MPCDiscrete_function_parameters.F_x0*x                  ...
            +    MPCDiscrete_function_parameters.F_du*u_prev    ...
    ); 
% 
    [a,b,c] =mpcActiveSetSolver(                                        ...                    
                                MPCDiscrete_function_parameters.Linv,                        ...                                    
                                F,                                      ...                    
                                MPCDiscrete_function_parameters.Ac,                          ...                                
                                new_b0,                                 ...                        
                                zeros(0,MPCDiscrete_function_parameters.N_prediction_steps), ...                                                        
                                zeros(0,1),                             ...                            
                                iA,                          ...                                
                                MPC_opt                                 ...                        
                            );
    new_iA = double(c); % Overwrite the old iA
    % u = a(1:length(a)/mpc_N_prediction_steps)
%     new_iA = zeros([80,1]); 
%     u = zeros([4,1]); 
    u = a(1:4);

== matlab function sandbox/LQG_controller/MPC_subsystem/LQG_controller/Controller_battery/MPCDiscreteAgnostic/MATLAB Function ==
  settings: updateMethod=DISCRETE  sampleTime=MPCDiscreteAgnostic_params.MPC_plant.Ts
  data: x input; ref input; u_prev input; iA input; u output size=4; MPCDiscreteAgnostic_function_parameters parameter; new_iA output size=size(MPCDiscreteAgnostic_function_parameters.iA)
function [u, new_iA] = fcn(x, ref, u_prev, iA,...
    MPCDiscreteAgnostic_function_parameters)


% Discrete_MPC_function_parameter
   % Might just set these manually... 
    MPC_opt = mpcActiveSetOptions;
    MPC_opt.IntegrityChecks = false;
    MPC_opt.UseHessianAsInput = false; 

%% Uncertain part
    new_b0 = MPCDiscreteAgnostic_function_parameters.b0;
    
    F = (                                           ...
                (MPCDiscreteAgnostic_function_parameters.F_y_ref* ref)           ...
            +    MPCDiscreteAgnostic_function_parameters.F_x0*x                  ...
            +    MPCDiscreteAgnostic_function_parameters.F_du*u_prev    ...
    ); 
% 
    [a,b,c] =mpcActiveSetSolver(                                        ...                    
                                MPCDiscreteAgnostic_function_parameters.Linv,                        ...                                    
                                F,                                      ...                    
                                MPCDiscreteAgnostic_function_parameters.Ac,                          ...                                
                                new_b0,                                 ...                        
                                zeros(0,MPCDiscreteAgnostic_function_parameters.N_prediction_steps), ...                                                        
                                zeros(0,1),                             ...                            
                                iA,                          ...                                
                                MPC_opt                                 ...                        
                            );
    new_iA = double(c); % Overwrite the old iA
    % u = a(1:length(a)/mpc_N_prediction_steps)
%     new_iA = zeros([80,1]); 
%     u = zeros([4,1]); 
    u = a(1:4);

== matlab function sandbox/LQG_controller/MPC_subsystem/LQG_controller/Controller_battery/MPCPseudoDiscrete/Cont mpc ==
  settings: updateMethod=CONTINUOUS  sampleTime=mpc_params.MPC_plant.Ts
  data: u output size=4; x input; ref input size=2; MPCPseudoDiscrete_function_parameters parameter
function u  = fcn(x, ref,...
    MPCPseudoDiscrete_function_parameters)


% Discrete_MPC_function_parameter
   % Might just set these manually... 
    MPC_opt = mpcActiveSetOptions;
    MPC_opt.IntegrityChecks = false;
    MPC_opt.UseHessianAsInput = false; 

%% Uncertain part
    new_b0 = MPCPseudoDiscrete_function_parameters.b0;
    
    F = (                                                                        ...
                (MPCPseudoDiscrete_function_parameters.F_y_ref* ref)           ...
            +    MPCPseudoDiscrete_function_parameters.F_x0*x                  ...
    ); 
% 
    [a,b,c] =mpcActiveSetSolver(                                        ...                    
                                MPCPseudoDiscrete_function_parameters.Linv,                        ...                                    
                                F,                                      ...                    
                                MPCPseudoDiscrete_function_parameters.Ac,                          ...                                
                                new_b0,                                 ...                        
                                zeros(0,MPCPseudoDiscrete_function_parameters.N_prediction_steps), ...                                                        
                                zeros(0,1),                             ...                            
                                zeros(size(new_b0)),                          ...                                
                                MPC_opt                                 ...                        
                            );

%     u = zeros([4,1]); 
    u = a(1:4);

== matlab function sandbox/LQG_controller/MPC_subsystem/LQG_controller/Controller_battery/MPCPseudoDiscreteAgnostic/Cont mpc ==
  settings: updateMethod=CONTINUOUS  sampleTime=mpc_params.MPC_plant.Ts
  data: u output size=4; x input; ref input size=2; MPCPseudoDiscreteAgnostic_function_parameters parameter
function u  = fcn(x, ref,...
    MPCPseudoDiscreteAgnostic_function_parameters)


% Discrete_MPC_function_parameter
   % Might just set these manually... 
    MPC_opt = mpcActiveSetOptions;
    MPC_opt.IntegrityChecks = false;
    MPC_opt.UseHessianAsInput = false; 

%% Uncertain part
    new_b0 = MPCPseudoDiscreteAgnostic_function_parameters.b0;
    
    F = (                                           ...
                (MPCPseudoDiscreteAgnostic_function_parameters.F_y_ref* ref)           ...
            +    MPCPseudoDiscreteAgnostic_function_parameters.F_x0*x                  ...
    ); 
% 
    [a,b,c] =mpcActiveSetSolver(                                        ...                    
                                MPCPseudoDiscreteAgnostic_function_parameters.Linv,                        ...                                    
                                F,                                      ...                    
                                MPCPseudoDiscreteAgnostic_function_parameters.Ac,                          ...                                
                                new_b0,                                 ...                        
                                zeros(0,MPCPseudoDiscreteAgnostic_function_parameters.N_prediction_steps), ...                                                        
                                zeros(0,1),                             ...                            
                                zeros(size(new_b0)),                          ...                                
                                MPC_opt                                 ...                        
                            );

%     u = zeros([4,1]); 
    u = a(1:4);

== matlab function sandbox/LQG_controller/MPC_subsystem/LQG_controller/Controller_battery/MPCDiscreteDiffIntegralAgnostic/MATLAB Function ==
  settings: updateMethod=DISCRETE  sampleTime=MPCDiscreteDiffIntegralAgnostic_params.MPC_plant.Ts
  data: x input size=19; ref input; u_prev input; iA input; u output size=4; MPCDiscreteDiffIntegralAgnostic_function_parameters parameter; new_iA output size=size(MPCDiscreteDiffIntegralAgnostic_function_parameters.iA)
function [u, new_iA] = fcn(x, ref, u_prev, iA,...
    MPCDiscreteDiffIntegralAgnostic_function_parameters)


% Discrete_MPC_function_parameter
   % Might just set these manually... 
    MPC_opt = mpcActiveSetOptions;
    MPC_opt.IntegrityChecks = false;
    MPC_opt.UseHessianAsInput = false; 

%% Uncertain part
    new_b0 = MPCDiscreteDiffIntegralAgnostic_function_parameters.b0;
    
    F = (                                           ...
                (MPCDiscreteDiffIntegralAgnostic_function_parameters.F_y_ref* ref)           ...
            +    MPCDiscreteDiffIntegralAgnostic_function_parameters.F_x0*x                  ...
            +    MPCDiscreteDiffIntegralAgnostic_function_parameters.F_du*u_prev    ...
    ); 
% 
    [a,b,c] =mpcActiveSetSolver(                                        ...                    
                                MPCDiscreteDiffIntegralAgnostic_function_parameters.Linv,                        ...                                    
                                F,                                      ...                    
                                MPCDiscreteDiffIntegralAgnostic_function_parameters.Ac,                          ...                                
                                new_b0,                                 ...                        
                                zeros(0,MPCDiscreteDiffIntegralAgnostic_function_parameters.N_prediction_steps), ...                                                        
                                zeros(0,1),                             ...                            
                                iA,                          ...                                
                                MPC_opt                                 ...                        
                            );
    new_iA = double(c); % Overwrite the old iA
    % u = a(1:length(a)/mpc_N_prediction_steps)
%     new_iA = zeros([80,1]); 
%     u = zeros([4,1]); 
    u = a(1:4);
